simulink model "zad_2_sch"  (R2022b)
settings: Solver=FixedStepAuto  StartTime=0.0  StopTime=0.5  FixedStep=0.0001  RelTol=1e-3
values from neighbouring files (symbols this model uses):
  a21 = 1/(2*m)*x30^2*FemP1/FemP2^2*exp(-x10/FemP2)    [zad_2.m]
  a23 = -1/(m)*x30*FemP1/FemP2*exp(-x10/FemP2)    [zad_2.m]
  a31 = 1/f1*exp(x10/f2)*(ki*u10+ci-x30)    [zad_2.m]
  a33 = -f2/f1*exp(x10/f2)    [zad_2.m]
  b31 = ki*f2/f1*exp(x10/f2)    [zad_2.m]
  g = 9.81    [zad_2.m]
  xd = d-bd    (= 0.0192)    [zad_2.m]
settings Model: Creator=AgraWoodAdmin  LastModifiedBy=AgraWoodAdmin
settings DebuggingCC: UnconnectedInputMsg=warning  UnconnectedOutputMsg=warning  UnconnectedLineMsg=warning
settings ModelReferenceCC: EnableRefExpFcnMdlSchedulingChecks=on
settings RTWCC: DLArmComputeVersion=19.05

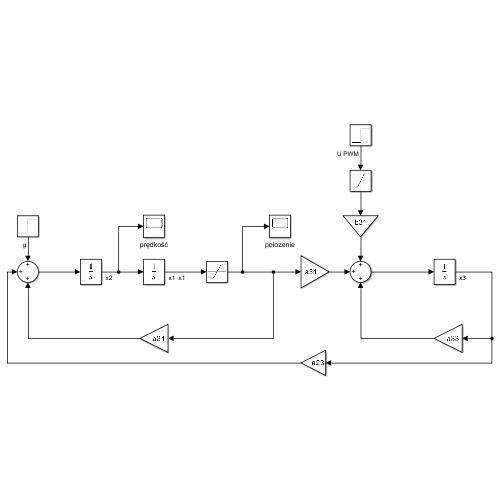
[thumbnail: Simulink's stored preview of the top-level diagram]
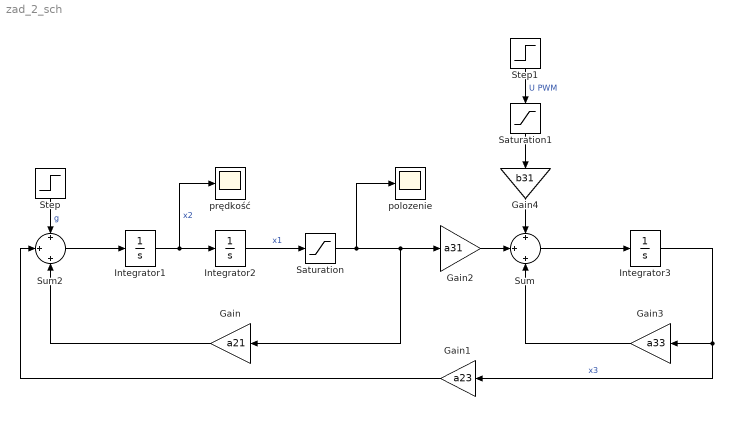
== system zad_2_sch ==
  Gain : Gain  Gain=a21
  Gain1 : Gain  Gain=a23
  Gain2 : Gain  Gain=a31
  Gain3 : Gain  Gain=a33
  Gain4 : Gain  Gain=b31
  Integrator1 : Integrator
  Integrator2 : Integrator  InitialCondition=xd
  Integrator3 : Integrator
  Saturation : Saturate  UpperLimit=xd  LowerLimit=0
  Saturation1 : Saturate  UpperLimit=1  LowerLimit=0
  Step : Step  Time=0  After=g  SampleTime=0
  Step1 : Step  Time=0  After=0.6  SampleTime=0
  Sum : Sum  Inputs=+|+|+
  Sum2 : Sum  Inputs=+|+|+
  polozenie : Scope
  prędkość : Scope
  wires:
  Sum2/1 -> Integrator1/1
  Sum/1 -> Integrator3/1
  Integrator1/1 -> prędkość/1, Integrator2/1  "x2"
  Integrator3/1 -> Gain3/1, Gain1/1  "x3"
  Gain/1 -> Sum2/3
  Gain1/1 -> Sum2/2
  Gain2/1 -> Sum/2
  Gain3/1 -> Sum/3
  Step1/1 -> Saturation1/1  "U PWM"
  Gain4/1 -> Sum/1
  Step/1 -> Sum2/1  "g"
  Integrator2/1 -> Saturation/1  "x1"
  Saturation1/1 -> Gain4/1
  Saturation/1 -> polozenie/1, Gain2/1, Gain/1
